simulink model "Fsw_model"  (R2017b)
settings: Solver=VariableStepAuto  StartTime=0.0  StopTime=1  RelTol=1e-3
settings Model: Creator=usama  LastModifiedBy=usama
settings DataIOCC: ReturnWorkspaceOutputs=on
settings DebuggingCC: UnconnectedInputMsg=none  UnconnectedOutputMsg=none  UnconnectedLineMsg=none
settings ModelReferenceCC: EnableRefExpFcnMdlSchedulingChecks=off
settings SFSimCC: SimUseLocalCustomCode=on
settings RTWCC: Description=Generic Real-Time Target  RTWUseLocalCustomCode=on

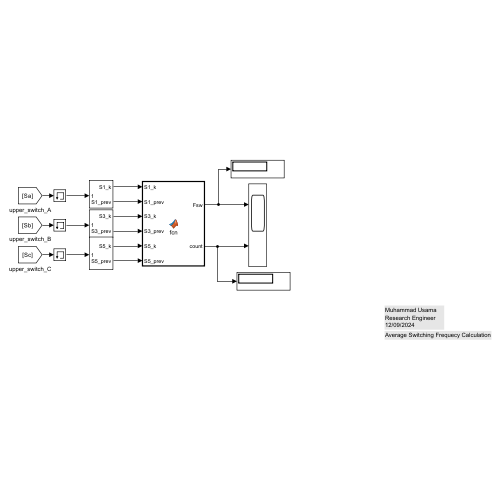
[thumbnail: Simulink's stored preview of the top-level diagram]
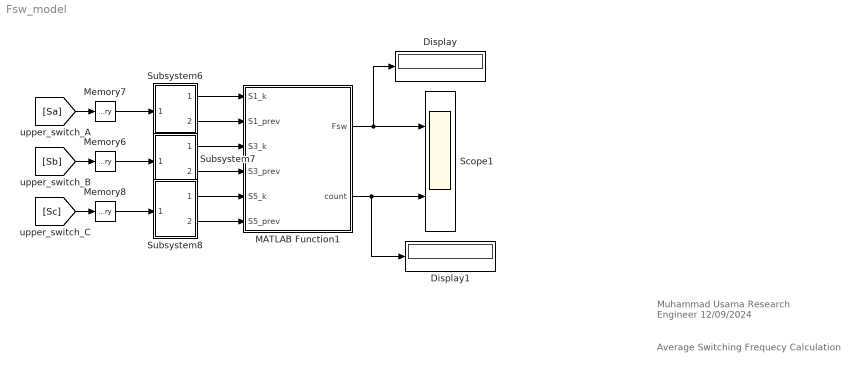
== system Fsw_model ==
  note: Average Switching Frequecy Calculation
  note: Muhammad Usama
      | Research Engineer
      | 12/09/2024
  Display : Display
  Display1 : Display
  MATLAB Function1 : MATLAB Function  TreatAsAtomicUnit=on
  Memory6 : Memory
  Memory7 : Memory
  Memory8 : Memory
  Scope1 : Scope  NumInputPorts=2
  Subsystem6 : Subsystem
  Subsystem7 : Subsystem
  Subsystem8 : Subsystem
  wires:
  Subsystem6/1(S1_k) -> MATLAB Function1/1(S1_k)
  Memory7/1 -> Subsystem6/1(In1)
  Memory6/1 -> Subsystem7/1(In1)
  [Sc] -> Memory8/1
  Memory8/1 -> Subsystem8/1(In1)
  Subsystem6/2(S1_prev) -> MATLAB Function1/2(S1_prev)
  [Sb] -> Memory6/1
  MATLAB Function1/1(Fsw) -> Scope1/1, Display/1
  [Sa] -> Memory7/1
  Subsystem7/1(S3_k) -> MATLAB Function1/3(S3_k)
  Subsystem7/2(S3_prev) -> MATLAB Function1/4(S3_prev)
  Subsystem8/1(S5_k) -> MATLAB Function1/5(S5_k)
  Subsystem8/2(S5_prev) -> MATLAB Function1/6(S5_prev)
  MATLAB Function1/2(count) -> Display1/1, Scope1/2

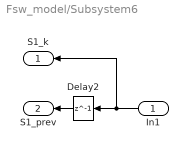
== system Fsw_model/Subsystem6 ==
  In1 : Inport
  Delay2 : Delay  DelayLength=1
  S1_k : Outport
  S1_prev : Outport  Port=2
  wires:
  Delay2/1 -> S1_prev/1
  In1/1 -> S1_k/1, Delay2/1

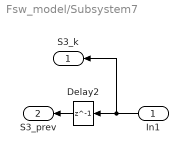
== system Fsw_model/Subsystem7 ==
  In1 : Inport
  Delay2 : Delay  DelayLength=1
  S3_k : Outport
  S3_prev : Outport  Port=2
  wires:
  In1/1 -> Delay2/1, S3_k/1
  Delay2/1 -> S3_prev/1

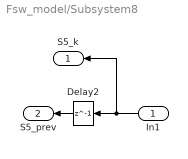
== system Fsw_model/Subsystem8 ==
  In1 : Inport
  Delay2 : Delay  DelayLength=1
  S5_k : Outport
  S5_prev : Outport  Port=2
  wires:
  Delay2/1 -> S5_prev/1
  In1/1 -> S5_k/1, Delay2/1

== matlab function Fsw_model/MATLAB Function1 ==
  data: S1_k input; Fsw output; S1_prev input; S3_k input; S3_prev input; S5_k input; S5_prev input; count output
function [Fsw ,count] = fcn(S1_k, S1_prev, S3_k, S3_prev, S5_k, S5_prev)

persistent switch_count1 sample_counter1 prev_avg_f_sw window_size

if isempty(switch_count1), switch_count1 = 0; end
if isempty(sample_counter1), sample_counter1 = 0; end
if isempty(prev_avg_f_sw), prev_avg_f_sw = 0; end
if isempty(window_size), window_size = 1000; end % Define window size (1000 samples)

    %% Calculate switching transitions
    S_k = [S1_k, S3_k, S5_k];
    S_prev = [S1_prev, S3_prev, S5_prev];
    Ts = 30e-6;

% Count switching events (sum(S_k ~= prev_S) gives the number of transitions)
    switch_count1 = switch_count1 + sum(S_k ~= S_prev);
    sample_counter1 = sample_counter1 + 1;

% Calculate average switching frequency over the window
if sample_counter1 >= window_size
    % Total time for the window
    window_time = window_size * Ts; % 1000 samples * 30e-6 = 0.03s
    % Average switching frequency
    avg_f_sw = switch_count1 / (3 * window_time); % Divide by 3 phases and window time
    prev_avg_f_sw = avg_f_sw;
    switch_count1 = 0; % Reset counter for the next window
    sample_counter1 = 0;
else
    avg_f_sw = prev_avg_f_sw; % Use previous average if window is not complete
end
Fsw = avg_f_sw ;
count = sample_counter1;
end
